simulink model "best_project_for_IG"  (R2023a)
settings: Solver=VariableStepAuto  StartTime=0.0  StopTime=t_final  RelTol=1e-3
StopFcn:
  | generateIndividualReport
values from neighbouring files (symbols this model uses):
  dq_0 = [0; 0; 0]    [Initialization.m]
  dt = 1.00e-03    (= 0.001)    [Initialization.m]
  initPosition = FwdKin(q_0)    [defineTrajectory.m]
undefined symbols (not defined in the file or in its folder): ikInitGuessSim, P1_R1_waypoints, P1_R1_waypointTimes, P1_R1_waypointVels, P2_R2_waypoints
libraries: simulink x6, robotcorelib x4, robotmaniplib x2
settings Model: Creator=lukasz  LastModifiedBy=lukasz

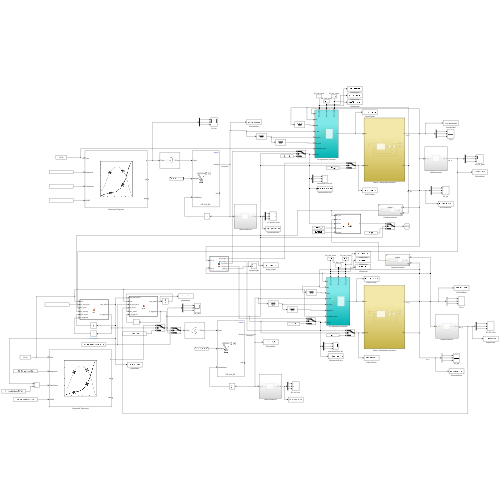
[thumbnail: Simulink's stored preview of the top-level diagram]
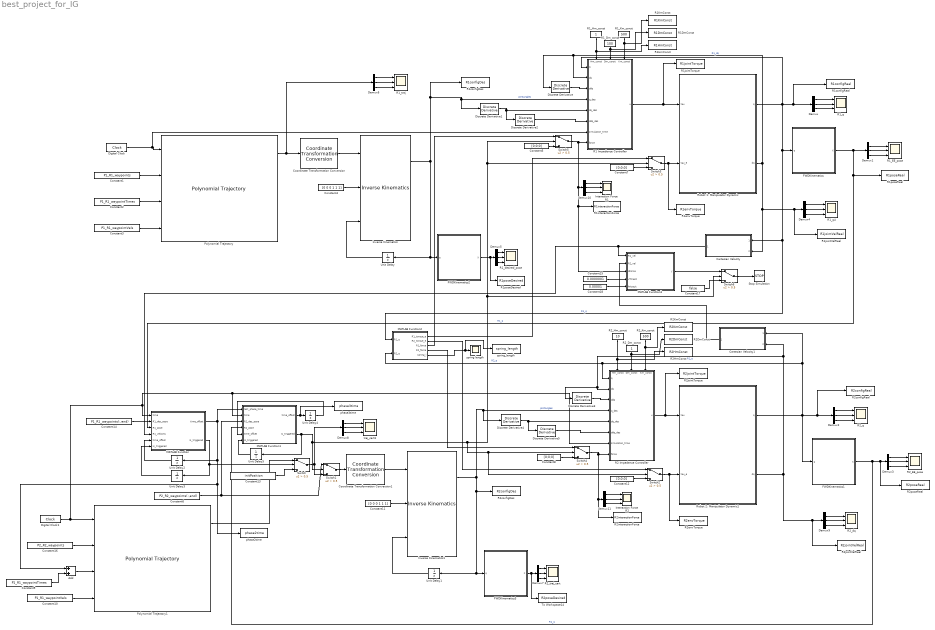
== system best_project_for_IG ==
  Add : Sum
  Cartesian Velocity : Subsystem  ReferencedSubsystem=dq2dp
  Cartesian Velocity1 : Subsystem  ReferencedSubsystem=dq2dp
  Constant1 : Constant  Value=P1_R1_waypoints  VectorParams1D=off  SampleTime=-1
  Constant10 : Constant  Value=P1_R1_waypointVels  VectorParams1D=off  SampleTime=-1
  Constant11 : Constant  Value=[0 0 0 1 1 1]  VectorParams1D=off
  Constant{5,7..8,12} (4 alike) : Constant  Value=[0;0;0]  VectorParams1D=off  SampleTime=-1
  Constant13 : Constant  Value=initPosition  VectorParams1D=off  SampleTime=-1
  Constant14 : Constant  Value=P1_R1_waypoints(:,end)  VectorParams1D=off  SampleTime=-1
  Constant15 : Constant  Value=0.0000001  VectorParams1D=off  SampleTime=-1
  Constant16 : Constant  Value=P2_R2_waypoints  VectorParams1D=off  SampleTime=-1
  Constant17 : Constant  Value=false  VectorParams1D=off  SampleTime=-1
  Constant18 : Constant  Value=0.00001  VectorParams1D=off  SampleTime=-1
  Constant2 : Constant  Value=P1_R1_waypointTimes  VectorParams1D=off  SampleTime=-1
  Constant3 : Constant  Value=P1_R1_waypointVels  VectorParams1D=off  SampleTime=-1
  Constant4 : Constant  Value=[0 0 0 1 1 1]  VectorParams1D=off
  Constant6 : Constant  Value=P2_R2_waypoints(:,end)  VectorParams1D=off  SampleTime=-1
  Constant9 : Constant  Value=P1_R1_waypointTimes  VectorParams1D=off  SampleTime=-1
  Coordinate Transformation Conversion : robotcorelib/Coordinate Transformation Conversion  InputRepresentation=Translation Vector  InputEulerSequence=ZYX  ShowTrVecInputPort=on  OutputRepresentation=Homogeneous Transformation  OutputEulerSequence=ZYX  ShowTrVecOutputPort=on  SimulateUsing=Code generation
  Coordinate Transformation Conversion1 : robotcorelib/Coordinate Transformation Conversion  InputRepresentation=Translation Vector  InputEulerSequence=ZYX  ShowTrVecInputPort=on  OutputRepresentation=Homogeneous Transformation  OutputEulerSequence=ZYX  ShowTrVecOutputPort=on  SimulateUsing=Code generation
  Demux{,1..11} (12 alike) : Demux  Outputs=3
  Digital Clock : DigitalClock  SampleTime=dt
  Digital Clock1 : DigitalClock  SampleTime=dt
  Discrete Derivative{,1..5} (6 alike) : simulink/Discrete/Discrete Derivative  gainval=1.0  ICPrevScaledInput=1  OutMin=[]  OutMax=[]  OutDataType=fixdt(1, 16)  OutScaling=2^-10  DoSatur=off
  FWDKinematics : Subsystem
  FWDKinematics1 : Subsystem
  FWDKinematics2 : Subsystem
  FWDKinematics3 : Subsystem
  Interaction Force R1 : Scope  NumInputPorts=3
  Interaction Force R2 : Scope  NumInputPorts=3
  Inverse Kinematics : robotmaniplib/Inverse Kinematics  RigidBodyTree=robot1  EndEffector=Link_EE  ShowInfo=on  SolverName=BFGS Gradient Projection  EnforceJointLimits=on  MaxIterations=1500  MaxTime=10  GradientTolerance=1e-7  SolutionTolerance=1e-6  StepTolerance=1e-14  ErrorChangeTolerance=1e-12  UseErrorDamping=on  DampingBias=0.0025  SimulateUsing=Code generation
  Inverse Kinematics1 : robotmaniplib/Inverse Kinematics  RigidBodyTree=robot1  EndEffector=Link_EE  ShowInfo=on  SolverName=BFGS Gradient Projection  EnforceJointLimits=on  MaxIterations=1500  MaxTime=10  GradientTolerance=1e-7  SolutionTolerance=1e-6  StepTolerance=1e-14  ErrorChangeTolerance=1e-12  UseErrorDamping=on  DampingBias=0.0025  SimulateUsing=Code generation
  MATLAB Function : MATLAB Function  TreatAsAtomicUnit=on
  MATLAB Function1 : MATLAB Function  TreatAsAtomicUnit=on
  MATLAB Function2 : MATLAB Function  TreatAsAtomicUnit=on
  MATLAB Function3 : MATLAB Function  TreatAsAtomicUnit=on
  Polynomial Trajectory : robotcorelib/Polynomial Trajectory  WaypointSource=External  Waypoints=[ 0, 2, 1, 5, 0; -1, 3, 1, 4, 4 ]  TimePoints=[ 0, 1, 2, 3, 4 ]  TimeInterval=[ 1, 4 ]  Method=Cubic Polynomial  ParameterSource=External  VelocityBoundaryCondition=zeros( 2, 5 )  AccelerationBoundaryCondition=zeros( 2, 5 )  SimulateUsing=Interpreted execution
  Polynomial Trajectory1 : robotcorelib/Polynomial Trajectory  WaypointSource=External  Waypoints=[ 0, 2, 1, 5, 0; -1, 3, 1, 4, 4 ]  TimePoints=[ 0, 1, 2, 3, 4 ]  TimeInterval=[ 1, 4 ]  Method=Cubic Polynomial  ParameterSource=External  VelocityBoundaryCondition=zeros( 2, 5 )  AccelerationBoundaryCondition=zeros( 2, 5 )  SimulateUsing=Interpreted execution
  R1 Impedence Controller : Subsystem
      settings: PortSchema="{\"entries\":[{\"content\":{\"sides\":[{\"content\":{\"connectorIds\":[\"In1\",\"In2\",\"In3\",\"In4\",\"In5\",\"In6\",\"In7\",\"In8\"]},\"type\":\"ConnectorPlacement.EquallySpacedRectSide\",\"uuid\":\"5dfe44b3-09a5-4539-84d6-5f1c3b4c2f7b\"},{\"content\":{\"connectorIds\":[\"Out1\"],\"side\":\"RIGHT\"},\"type\":\"ConnectorPlacement.EquallySpacedRectSide\",\"uuid\":\"14568bd5-ea33-4e20-b738-babf2c0b76a3\"},{\"content\":{\"connectorIds\":[\"In9\",\"In10\",\"In11\"],\"side\":\"TOP\"},\"type\":\"ConnectorPlacement.EquallySpacedRectSide\",\"uuid\":\"79ac3c01-1ab3-40ba-b47a-1253ed034708\"}]},\"type\":\"ConnectorPlacement.EquallySpacedConnector\",\"uuid\":\"3e0c5e05-24f3-4436-a36d-058567bfa2f1\"}],\"packageUris\":[\"http://schema.mathworks.com/mf0/Connector/R2020b\"],\"version\":\"1.0\"}"
  R1DmConst : ToWorkspace  VariableName=R1DmConst  SaveFormat=Timeseries  SampleTime=-1
  R1HmConst : ToWorkspace  VariableName=R1HmConst  SaveFormat=Timeseries  SampleTime=-1
  R1KmConst : ToWorkspace  VariableName=R1KmConst  SaveFormat=Timeseries  SampleTime=-1
  R1_Dm_const : Constant  Value=100  VectorParams1D=off  SampleTime=-1
  R1_EE_pose : Scope  NumInputPorts=3
  R1_Hm_const : Constant  VectorParams1D=off  SampleTime=-1
  R1_Km_const : Constant  Value=500  VectorParams1D=off  SampleTime=-1
  R1_desired_pose : Scope  NumInputPorts=3
  R1_q : Scope  NumInputPorts=3
  R1_q4 : Scope  NumInputPorts=3
  R1_traj : Scope  NumInputPorts=3
  R1configDes : ToWorkspace  VariableName=R1configDes  SaveFormat=Timeseries  SampleTime=-1
  R1configReal : ToWorkspace  VariableName=R1configReal  SaveFormat=Timeseries  SampleTime=-1
  R1envTorque : ToWorkspace  VariableName=R1envTorque  SaveFormat=Timeseries  SampleTime=-1
  R1interactionForce : ToWorkspace  VariableName=R1interactionForce  SaveFormat=Timeseries  SampleTime=-1
  R1jointTorque : ToWorkspace  VariableName=R1jointTorque  SaveFormat=Timeseries  SampleTime=-1
  R1jointVelReal : ToWorkspace  VariableName=R1jointVelReal  SaveFormat=Timeseries  SampleTime=-1
  R1poseDesired : ToWorkspace  VariableName=R1poseDesired  SaveFormat=Timeseries  SampleTime=-1
  R1poseReal : ToWorkspace  VariableName=R1poseReal  SaveFormat=Timeseries  SampleTime=-1
  R2 Impedence Controller : Subsystem
      settings: PortSchema="{\"entries\":[{\"content\":{\"sides\":[{\"content\":{\"connectorIds\":[\"In1\",\"In2\",\"In3\",\"In4\",\"In5\",\"In6\",\"In7\",\"In8\"]},\"type\":\"ConnectorPlacement.EquallySpacedRectSide\",\"uuid\":\"5dfe44b3-09a5-4539-84d6-5f1c3b4c2f7b\"},{\"content\":{\"connectorIds\":[\"Out1\"],\"side\":\"RIGHT\"},\"type\":\"ConnectorPlacement.EquallySpacedRectSide\",\"uuid\":\"14568bd5-ea33-4e20-b738-babf2c0b76a3\"},{\"content\":{\"connectorIds\":[\"In9\",\"In10\",\"In11\"],\"side\":\"TOP\"},\"type\":\"ConnectorPlacement.EquallySpacedRectSide\",\"uuid\":\"79ac3c01-1ab3-40ba-b47a-1253ed034708\"}]},\"type\":\"ConnectorPlacement.EquallySpacedConnector\",\"uuid\":\"3e0c5e05-24f3-4436-a36d-058567bfa2f1\"}],\"packageUris\":[\"http://schema.mathworks.com/mf0/Connector/R2020b\"],\"version\":\"1.0\"}"
  R2DmConst : ToWorkspace  VariableName=R2DmConst  SaveFormat=Timeseries  SampleTime=-1
  R2HmConst : ToWorkspace  VariableName=R2HmConst  SaveFormat=Timeseries  SampleTime=-1
  R2KmConst : ToWorkspace  VariableName=R2KmConst  SaveFormat=Timeseries  SampleTime=-1
  R2_Dm_const : Constant  VectorParams1D=off  SampleTime=-1
  R2_EE_pose : Scope  NumInputPorts=3
  R2_Hm_const : Constant  Value=10  VectorParams1D=off  SampleTime=-1
  R2_Km_const : Constant  Value=500  VectorParams1D=off  SampleTime=-1
  R2_dq : Scope  NumInputPorts=3
  R2_q : Scope  NumInputPorts=3
  R2_traj_cart : Scope  NumInputPorts=3
  R2configDes : ToWorkspace  VariableName=R2configDes  SaveFormat=Timeseries  SampleTime=-1
  R2configReal : ToWorkspace  VariableName=R2configReal  SaveFormat=Timeseries  SampleTime=-1
  R2envTorque : ToWorkspace  VariableName=R2envTorque  SaveFormat=Timeseries  SampleTime=-1
  R2interactionForce : ToWorkspace  VariableName=R2interactionForce  SaveFormat=Timeseries  SampleTime=-1
  R2jointTorque : ToWorkspace  VariableName=R2jointTorque  SaveFormat=Timeseries  SampleTime=-1
  R2jointVelReal : ToWorkspace  VariableName=R2jointVelReal  SaveFormat=Timeseries  SampleTime=-1
  R2poseReal : ToWorkspace  VariableName=R2poseReal  SaveFormat=Timeseries  SampleTime=-1
  Robot 1: Manipulator Dynamic : Subsystem
  Robot 2: Manipulator Dynamic1 : Subsystem
  Stop Simulation : Stop
  Switch{,1..6} (7 alike) : Switch  Criteria=u2 > Threshold  Threshold=0.5  SaturateOnIntegerOverflow=off  InputSameDT=off
  To Workspace14 : ToWorkspace  VariableName=R2poseDesired  SaveFormat=Timeseries  SampleTime=-1
  Unit Delay : UnitDelay  InitialCondition=ikInitGuessSim  SampleTime=-1  HasFrameUpgradeWarning=on
  Unit Delay1 : UnitDelay  InitialCondition=ikInitGuessSim  SampleTime=-1  HasFrameUpgradeWarning=on
  Unit Delay{2..5} (4 alike) : UnitDelay  SampleTime=-1  HasFrameUpgradeWarning=on
  phase2time : ToWorkspace  VariableName=phase2time  SaveFormat=Timeseries  SampleTime=-1
  phase3time : ToWorkspace  VariableName=phase3time  SaveFormat=Timeseries  SampleTime=-1
  spring length : Scope
  spring_length : ToWorkspace  VariableName=spring_length  SaveFormat=Timeseries  SampleTime=-1
  traj_cart3 : Scope  NumInputPorts=3
  wires:
  Demux/3 -> R1_q/3
  Robot 1: Manipulator Dynamic/1(q) -> R1 Impedence Controller/1(q), FWDKinematics/1(q), MATLAB Function2/1(R1_q), Cartesian Velocity/1, R1configReal/1, Demux/1  "R1_q"
  Demux/1 -> R1_q/1
  Demux/2 -> R1_q/2
  Constant1/1 -> Polynomial Trajectory/2
  Inverse Kinematics/1 -> FWDKinematics2/1(q), Unit Delay/1, R1configDes/1, Discrete Derivative1/1, R1 Impedence Controller/4(q_des)  "jointAngles"
  Unit Delay/1 -> Inverse Kinematics/3
  Constant4/1 -> Inverse Kinematics/2
  Digital Clock/1 -> R1 Impedence Controller/7(simulation_time), Polynomial Trajectory/1
  Constant3/1 -> Polynomial Trajectory/4
  Constant2/1 -> Polynomial Trajectory/3
  Demux1/1 -> R1_EE_pose/1
  Demux1/2 -> R1_EE_pose/2
  Demux1/3 -> R1_EE_pose/3
  FWDKinematics/1(X) -> R1poseReal/1, MATLAB Function/3(R1_pose), Demux1/1  "R1_q"
  Demux3/2 -> R2_EE_pose/2
  Demux2/3 -> R2_q/3
  Demux3/1 -> R2_EE_pose/1
  Demux2/1 -> R2_q/1
  Demux2/2 -> R2_q/2
  Demux3/3 -> R2_EE_pose/3
  Robot 2: Manipulator Dynamic1/1(q) -> Cartesian Velocity1/1, R2 Impedence Controller/1(q), MATLAB Function2/2(R2_q), FWDKinematics1/1(q), R2configReal/1, Demux2/1  "R2_q"
  FWDKinematics1/1(X) -> MATLAB Function1/4(R2_pose), R2poseReal/1, Demux3/1  "R1_q"
  Demux4/1 -> R1_q4/1
  Demux4/2 -> R1_q4/2
  Demux4/3 -> R1_q4/3
  Robot 1: Manipulator Dynamic/2(dq) -> Discrete Derivative/1, R1 Impedence Controller/2(dq), Cartesian Velocity/2, R1jointVelReal/1, Demux4/1  "R1_dq"
  Demux5/1 -> R1_desired_pose/1
  Demux5/2 -> R1_desired_pose/2
  Demux5/3 -> R1_desired_pose/3
  FWDKinematics2/1(X) -> R1poseDesired/1, Demux5/1
  Demux6/3 -> R1_traj/3
  Demux6/1 -> R1_traj/1
  Demux6/2 -> R1_traj/2
  Polynomial Trajectory/1 -> Coordinate Transformation Conversion/1, Demux6/1
  Coordinate Transformation Conversion/1 -> Inverse Kinematics/1
  R1 Impedence Controller/1(u) -> R1jointTorque/1, Robot 1: Manipulator Dynamic/1(tau)
  Discrete Derivative/1 -> R1 Impedence Controller/3(ddq)
  Discrete Derivative1/1 -> Discrete Derivative2/1, R1 Impedence Controller/5(dq_des)
  Discrete Derivative2/1 -> R1 Impedence Controller/6(ddq_des)
  Unit Delay1/1 -> Inverse Kinematics1/3
  Digital Clock1/1 -> MATLAB Function/1(time), R2 Impedence Controller/7(simulation_time), MATLAB Function1/2(time), Polynomial Trajectory1/1
  Demux7/1 -> R2_traj_cart/1
  Discrete Derivative4/1 -> R2 Impedence Controller/5(dq_des), Discrete Derivative5/1
  Constant16/1 -> Polynomial Trajectory1/2
  Inverse Kinematics1/1 -> R2configDes/1, FWDKinematics3/1(q), Unit Delay1/1, R2 Impedence Controller/4(q_des), Discrete Derivative4/1  "jointAngles"
  Discrete Derivative5/1 -> R2 Impedence Controller/6(ddq_des)
  Demux7/3 -> R2_traj_cart/3
  R2 Impedence Controller/1(u) -> R2jointTorque/1, Robot 2: Manipulator Dynamic1/1(tau)
  Demux7/2 -> R2_traj_cart/2
  FWDKinematics3/1(X) -> To Workspace14/1, Demux7/1
  Discrete Derivative3/1 -> R2 Impedence Controller/3(ddq)
  Demux8/3 -> traj_cart3/3
  Demux8/2 -> traj_cart3/2
  Constant11/1 -> Inverse Kinematics1/2
  Constant10/1 -> Polynomial Trajectory1/4
  Demux8/1 -> traj_cart3/1
  Coordinate Transformation Conversion1/1 -> Inverse Kinematics1/1
  Demux9/3 -> R2_dq/3
  Demux9/1 -> R2_dq/1
  Robot 2: Manipulator Dynamic1/2(dq) -> R2jointVelReal/1, Demux9/1, R2 Impedence Controller/2(dq), Discrete Derivative3/1, Cartesian Velocity1/2  "R1_q"
  Demux9/2 -> R2_dq/2
  Switch/1 -> Switch1/3, Demux8/1
  Polynomial Trajectory1/1 -> Switch/1
  Constant13/1 -> Switch/3
  Unit Delay2/1 -> MATLAB Function/5("time_offset ")
  Add/1 -> Polynomial Trajectory1/3
  Constant9/1 -> Add/2
  Unit Delay3/1 -> MATLAB Function/6("is_triggered ")
  MATLAB Function/2(is_triggered) -> Switch/2, Unit Delay3/1
  MATLAB Function/1(time_offset) -> phase2time/1, Add/1, Unit Delay2/1, MATLAB Function1/1(last_phase_time)
  Constant14/1 -> MATLAB Function/2(R1_des_pose)
  Cartesian Velocity/1 -> MATLAB Function/4(R1_velocity), MATLAB Function3/1(R1_vel)
  Switch1/1 -> Coordinate Transformation Conversion1/1
  MATLAB Function1/2(is_triggered) -> Unit Delay5/1, Switch5/2, Switch3/2, Switch6/2, Switch2/2, Switch4/2, Switch1/2
  MATLAB Function1/1(time_offset) -> phase3time/1, Unit Delay4/1
  Unit Delay4/1 -> MATLAB Function1/5("time_offset ")
  Unit Delay5/1 -> MATLAB Function1/6("is_triggered ")
  Constant6/1 -> Switch1/1, MATLAB Function1/3(R2_des_pose)
  Switch2/1 -> R2envTorque/1, Robot 2: Manipulator Dynamic1/2(tau_e)
  Switch3/1 -> R1envTorque/1, Robot 1: Manipulator Dynamic/2(tau_e)
  Constant5/1 -> Switch5/3
  Constant7/1 -> Switch3/3
  Constant8/1 -> Switch4/3
  Constant12/1 -> Switch2/3
  MATLAB Function2/4(R2_force) -> Switch4/1
  MATLAB Function2/2(R2_torque_e) -> Switch2/1
  MATLAB Function2/1(R1_torque_e) -> Switch3/1
  MATLAB Function2/3(R1_force) -> Switch5/1
  Demux10/1 -> Interaction Force R1/1
  Demux10/2 -> Interaction Force R1/2
  Demux10/3 -> Interaction Force R1/3
  Switch5/1 -> MATLAB Function3/3(dForce), R1interactionForce/1, Demux10/1, R1 Impedence Controller/8(force)
  Demux11/3 -> Interaction Force R2/3
  Demux11/1 -> Interaction Force R2/1
  Switch4/1 -> R2 Impedence Controller/8(force), R2interactionForce/1, Demux11/1
  Demux11/2 -> Interaction Force R2/2
  MATLAB Function2/5(spring_l) -> spring_length/1, spring length/1
  R1_Hm_const/1 -> R1 Impedence Controller/9(Hm_const), R1HmConst/1
  R1_Dm_const/1 -> R1 Impedence Controller/10(Dm_const), R1DmConst/1
  R1_Km_const/1 -> R1 Impedence Controller/11(Km_const), R1KmConst/1
  R2_Km_const/1 -> R2KmConst/1, R2 Impedence Controller/11(Km_const)
  R2_Hm_const/1 -> R2HmConst/1, R2 Impedence Controller/9(Hm_const)
  R2_Dm_const/1 -> R2 Impedence Controller/10(Dm_const), R2DmConst/1
  MATLAB Function3/1(y) -> Switch6/1
  Switch6/1 -> Stop Simulation/1
  Constant17/1 -> Switch6/3
  Cartesian Velocity1/1 -> MATLAB Function3/2(R2_vel)
  Constant15/1 -> MATLAB Function3/4(vThresh)
  Constant18/1 -> MATLAB Function3/5(fThresh)

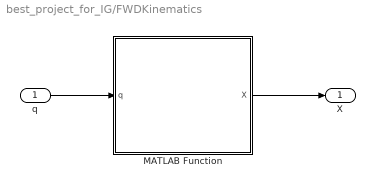
== system best_project_for_IG/FWDKinematics ==
  q : Inport
  MATLAB Function : MATLAB Function  TreatAsAtomicUnit=on
  X : Outport
  wires:
  MATLAB Function/1(X) -> X/1
  q/1 -> MATLAB Function/1(q)

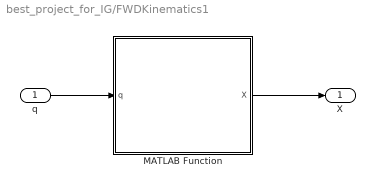
== system best_project_for_IG/FWDKinematics1 ==
  q : Inport
  MATLAB Function : MATLAB Function  TreatAsAtomicUnit=on
  X : Outport
  wires:
  MATLAB Function/1(X) -> X/1
  q/1 -> MATLAB Function/1(q)

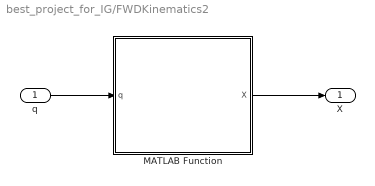
== system best_project_for_IG/FWDKinematics2 ==
  q : Inport
  MATLAB Function : MATLAB Function  TreatAsAtomicUnit=on
  X : Outport
  wires:
  MATLAB Function/1(X) -> X/1
  q/1 -> MATLAB Function/1(q)

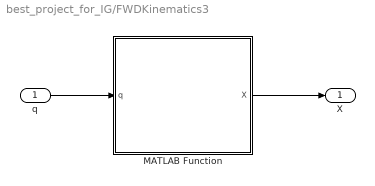
== system best_project_for_IG/FWDKinematics3 ==
  q : Inport
  MATLAB Function : MATLAB Function  TreatAsAtomicUnit=on
  X : Outport
  wires:
  MATLAB Function/1(X) -> X/1
  q/1 -> MATLAB Function/1(q)

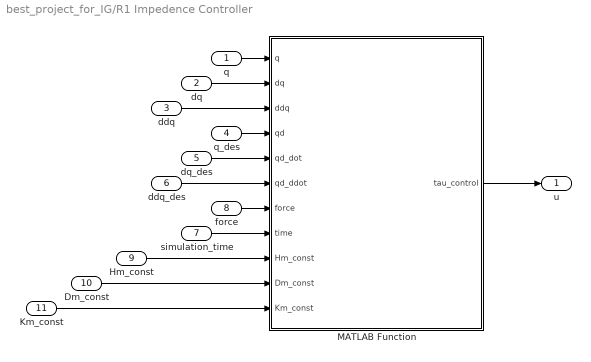
== system best_project_for_IG/R1 Impedence Controller ==
  q : Inport
  dq : Inport  Port=2
  ddq : Inport  Port=3
  q_des : Inport  Port=4
  dq_des : Inport  Port=5
  ddq_des : Inport  Port=6
  simulation_time : Inport  Port=7
  force : Inport  Port=8
  Hm_const : Inport  Port=9
  Dm_const : Inport  Port=10
  Km_const : Inport  Port=11
  MATLAB Function : MATLAB Function  TreatAsAtomicUnit=on
  u : Outport
  wires:
  dq/1 -> MATLAB Function/2(dq)
  MATLAB Function/1(tau_control) -> u/1
  q_des/1 -> MATLAB Function/4(qd)
  q/1 -> MATLAB Function/1(q)
  ddq_des/1 -> MATLAB Function/6(qd_ddot)
  dq_des/1 -> MATLAB Function/5(qd_dot)
  simulation_time/1 -> MATLAB Function/8(time)
  ddq/1 -> MATLAB Function/3(ddq)
  force/1 -> MATLAB Function/7(force)
  Hm_const/1 -> MATLAB Function/9(Hm_const)
  Dm_const/1 -> MATLAB Function/10(Dm_const)
  Km_const/1 -> MATLAB Function/11(Km_const)

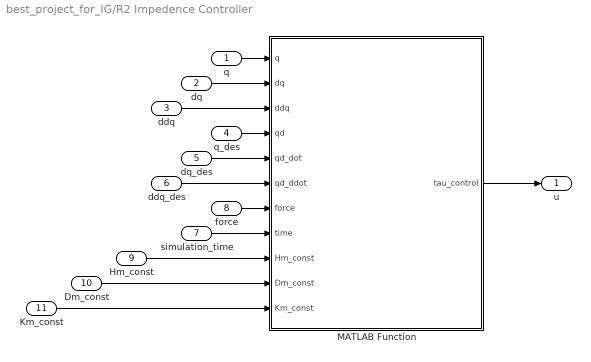
== system best_project_for_IG/R2 Impedence Controller ==
  q : Inport
  dq : Inport  Port=2
  ddq : Inport  Port=3
  q_des : Inport  Port=4
  dq_des : Inport  Port=5
  ddq_des : Inport  Port=6
  simulation_time : Inport  Port=7
  force : Inport  Port=8
  Hm_const : Inport  Port=9
  Dm_const : Inport  Port=10
  Km_const : Inport  Port=11
  MATLAB Function : MATLAB Function  TreatAsAtomicUnit=on
  u : Outport
  wires:
  dq/1 -> MATLAB Function/2(dq)
  MATLAB Function/1(tau_control) -> u/1
  q_des/1 -> MATLAB Function/4(qd)
  q/1 -> MATLAB Function/1(q)
  ddq_des/1 -> MATLAB Function/6(qd_ddot)
  dq_des/1 -> MATLAB Function/5(qd_dot)
  simulation_time/1 -> MATLAB Function/8(time)
  ddq/1 -> MATLAB Function/3(ddq)
  force/1 -> MATLAB Function/7(force)
  Hm_const/1 -> MATLAB Function/9(Hm_const)
  Dm_const/1 -> MATLAB Function/10(Dm_const)
  Km_const/1 -> MATLAB Function/11(Km_const)

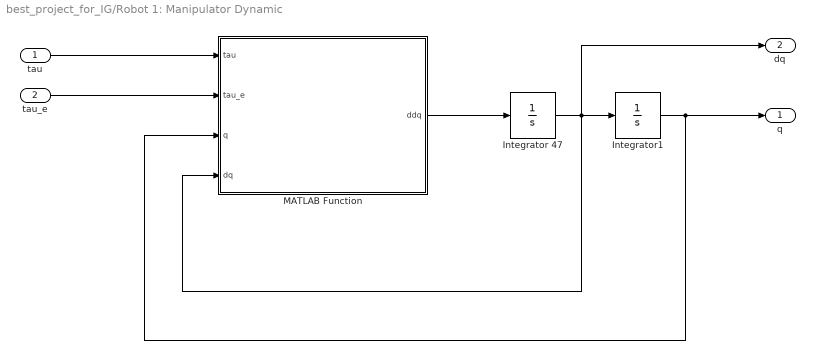
== system best_project_for_IG/Robot 1: Manipulator Dynamic ==
  tau : Inport
  tau_e : Inport  Port=2
  Integrator 47 : Integrator  InitialCondition=dq_0
  Integrator1 : Integrator  InitialCondition=ikInitGuessSim
  MATLAB Function : MATLAB Function  TreatAsAtomicUnit=on
  q : Outport
  dq : Outport  Port=2
  wires:
  MATLAB Function/1(ddq) -> Integrator 47/1
  tau/1 -> MATLAB Function/1(tau)
  tau_e/1 -> MATLAB Function/2(tau_e)
  Integrator1/1 -> q/1, MATLAB Function/3(q)
  Integrator 47/1 -> dq/1, MATLAB Function/4(dq), Integrator1/1

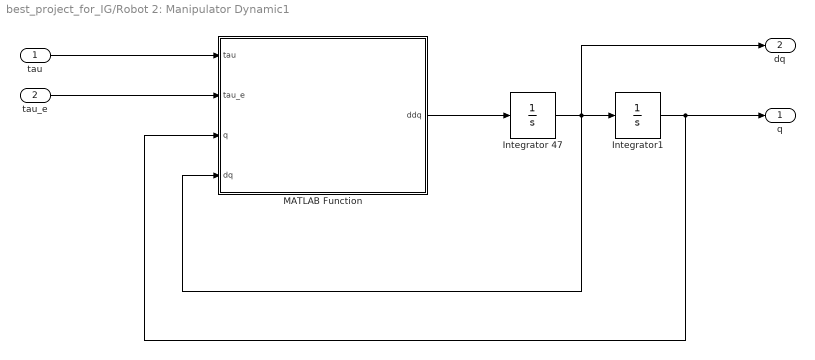
== system best_project_for_IG/Robot 2: Manipulator Dynamic1 ==
  tau : Inport
  tau_e : Inport  Port=2
  Integrator 47 : Integrator  InitialCondition=dq_0
  Integrator1 : Integrator  InitialCondition=ikInitGuessSim
  MATLAB Function : MATLAB Function  TreatAsAtomicUnit=on
  q : Outport
  dq : Outport  Port=2
  wires:
  MATLAB Function/1(ddq) -> Integrator 47/1
  tau/1 -> MATLAB Function/1(tau)
  tau_e/1 -> MATLAB Function/2(tau_e)
  Integrator1/1 -> q/1, MATLAB Function/3(q)
  Integrator 47/1 -> dq/1, MATLAB Function/4(dq), Integrator1/1

== matlab function best_project_for_IG/MATLAB Function1 ==
  data: last_phase_time input; time input; R2_des_pose input; R2_pose input; time_offset input; time_offset output; is_triggered input; is_triggered output
function [time_offset, is_triggered] = fcn(last_phase_time, time, R2_des_pose, R2_pose, time_offset, is_triggered)

x_trigger = R2_des_pose(1);
current_x = R2_pose(1);

if ((time > (last_phase_time+6)) && ...
        current_x >= x_trigger && (is_triggered==0))
    time_offset = time;
    is_triggered = 1;
end

== matlab function best_project_for_IG/R1 Impedence Controller/MATLAB Function ==
  data: q input; dq input; ddq input; tau_control output; qd input; qd_dot input; qd_ddot input; force input; time input; Hm_const input; Dm_const input; Km_const input
function tau_control = fcn(q, dq, ddq, qd, qd_dot, qd_ddot,force,...
                           time, Hm_const, Dm_const, Km_const)
% reset first qd_ddot
if (time < 0.003)
    qd_ddot = [0;0;0];
    qd_dot = [0;0;0];
    ddq = [0;0;0];
end


%% Joint Space variables

q1 = q(1);
q2 = q(2);
q3 = q(3);

dq1 = dq(1);
dq2 = dq(2);
dq3 = dq(3);

%% general physical parameters

l1 = 0.6731;
l2 = 0.432;
l3 = 0.434;
lc2 = 0.216;
lc3 = 0.164;
m2 = 15.46;
m3 = 9.55;
J = 0.302;

%% Inertia Matrix Parameters

J1 = m3 * lc3^2;
J12 = (m2 * lc2^2) + (m3 * l2^2);
J13 = l2 * lc3 * m3;


h11 = J + J1 * (sin(q2 + q3))^2 + J12 * (cos(q2))^2 + 2 * J13 * cos(q2) * sin(q2+q3);
h22 = J1 + J12 + 2 * J13 * sin(q3);
h23 = J1 + J13 * sin(q3);
h32 = h23;
h33 = J1;

H = [h11, 0 ,0 ;
    0 , h22, h23;
    0 , h32, h33];

%% Coriolis Matrix Parameters

c12_1 = J1 * sin(2 * (q1 + q2)) - J12 * sin(2 * q2) + 2 * J13 * cos(2 * q2 +q3);
c13_1 = J1 * sin(2 * (q2 + q3)) + 2 * J13 * cos(q2) * cos(q2 + q3);
c11_2 = (1/2) * (-J1 * sin(2 * (q2 + q3)) + J12 * sin(2 * q2) - 2 * J13 * cos(2 * q2 + q3));
c22_2 = 2 * J13 * cos(q3);
c23_2 = J13 * cos(q3);
c22_3 = -J13 * cos(q3) * dq2;
c11_3 = (-1/2) * (J1 * sin(2 * (q2 + q3)) + J13 * cos(q2) * cos(q2 + q3));

C = [0, c12_1 * dq1, c13_1 * dq3;
    c11_2 * dq1, 0 , c22_2 * dq2 + c23_2 * dq3;
    c11_3 * dq1, c22_3 * dq2, 0];

%% Vector of Potential Forces Parameters

g = 9.81;

g21 = -g * (lc3 * m3 * sin(q2 + q3) + lc2 * m2 * cos(q2) + l2 * m3 * cos(q2));
g31 = -g * (lc3 * m3 * sin(q2 + q3));

G = [0;
    g21;
    g31];


%% get Jacobians
J = jacobian(q);
dJ = dJacobian(q,dq);

%% convert to task space
Hp = inv(J') * H * inv(J);
Cp = inv(J') * C * inv(J) - Hp * dJ * inv(J);
Gp = inv(J') * G;

%% desired behaviour
Hm = Hm_const*eye(3,3);
Dm = Dm_const*eye(3,3);
Km = Km_const*eye(3,3);

%% get postion and its derivs
p = fwdKin(q);
dp = J * dq;
ddp = dJ * dq + J * ddq;

%% get desired postion and its derivs
pd = fwdKin(qd);
pd_dot = jacobian(qd) * qd_dot;
pd_ddot = dJacobian(qd,qd_dot) * qd_dot + jacobian(qd) * qd_ddot;

%% define u note

u_note = pd_ddot + inv(Hm) * (Dm * (pd_dot-dp) + Km*(pd - p) + force);
inv_hm = inv(Hm);
%% define tau_control

tau_control = J' * (Hp * u_note + Cp * dp + Gp - force);


function [X] = fwdKin(Q)
    s1 = sin(Q(1, :));
    c1 = cos(Q(1, :));
    s2 = sin(Q(2, :));
    c2 = cos(Q(2, :));
    s23 = sin(Q(2, :) + Q(3, :));
    c23 = cos(Q(2, :) + Q(3, :));
    l = [0.6731; 0.432; 0.434];
    
    X = zeros(3,1);
    X(1, :) = c1.*(l(2)*c2 + l(3)*s23);
    X(2, :) = s1.*(l(2)*c2 + l(3)*s23);
    X(3, :) = l(1) - l(2)*s2 + l(3)*c23;

function dJ = dJacobian(Q, dQ)
    l = [0.6731; 0.432; 0.434];
    s1 = sin(Q(1));
    c1 = cos(Q(1));
    s2 = sin(Q(2));
    c2 = cos(Q(2));
    s23 = sin(Q(2) + Q(3));
    c23 = cos(Q(2) + Q(3));

    % dJi derivative of each element of Jacobian wrt i-th variable            
    %--- 1 ---
    dJ1 = [-c1*(l(2)*c2 + l(3)*s23), -s1*(-l(2)*s2 + l(3)*c23), -l(3)*s1*c23;...
           -s1*(l(2)*c2 + l(3)*s23),  c1*(-l(2)*s2 + l(3)*c23),  l(3)*c1*c23;...
           0, 0, 0];
    %--- 2 ---   
    dJ2 = [-s1*(-l(2)*s2 + l(3)*c23), -c1*(l(2)*c2 + l(3)*s23), -l(3)*c1*s23;...
            c1*(-l(2)*s2 + l(3)*c23), -s1*(l(2)*c2 + l(3)*s23), -l(3)*s1*s23;...
            0, l(2)*s2 - l(3)*c23, -l(3)*c23];

    %--- 3 ---
    dJ3 = -l(3)*[ s1*c23, c1*s23, c1*s23;...
                 -c1*c23, s1*s23, s1*s23;...
                 0, c23, c23];
    %--- dJ ---
    dJ = dJ1*dQ(1) + dJ2*dQ(2) + dJ3*dQ(3);

function [J] = jacobian(q)

l = [0.6731; 0.432; 0.434];
s1 = sin(q(1));
c1 = cos(q(1));
s2 = sin(q(2));
c2 = cos(q(2));
s23 = sin(q(2) + q(3));
c23 = cos(q(2) + q(3));

J = zeros(3,3);

J(1, 1) = -s1*( l(2)*c2 + l(3)*s23);
J(1, 2) =  c1*(-l(2)*s2 + l(3)*c23);
J(1, 3) = l(3)*c1*c23;

J(2, 1) = c1*( l(2)*c2 + l(3)*s23);
J(2, 2) = s1*(-l(2)*s2 + l(3)*c23);
J(2, 3) = l(3)*s1*c23;

J(3, 2) = -l(2)*c2 - l(3)*s23;
J(3, 3) = -l(3)*s23;

== matlab function best_project_for_IG/MATLAB Function3 ==
  data: R1_vel input; y output; R2_vel input; dForce input; vThresh input; fThresh input
function y = stopCondition(R1_vel, R2_vel, dForce, vThresh, fThresh)

if (norm(R1_vel) <= vThresh) && ...
   (norm(R2_vel) <= vThresh) && ...
   (norm(dForce) <= fThresh)
    y = true;
else
    y = false;
end

end

== matlab function best_project_for_IG/MATLAB Function2 ==
  data: R1_q input; R1_torque_e output; R2_q input; R2_torque_e output; R1_force output; R2_force output; spring_l output
function [R1_torque_e, R2_torque_e, R1_force, R2_force, spring_l] = fcn(R1_q, R2_q)

uncompressed_spring_len = 0.2;

R1_pose = fwdKin(R1_q);
R2_pose = fwdKin(R2_q);

% transforms and rod definition
rod_length = [0.20;0;0]; % meters
R1_T_R2 = [-1,  0,  0, 0.7395*2 + rod_length(1);
            0, -1,  0,                            0;
            0,  0,  1,                            0;
            0,  0,  0,                            1];

R2_T_R1 = [-1,  0,  0, 0.7395*2 + rod_length(1);
            0, -1,  0,                            0;
            0,  0,  1,                            0;
            0,  0,  0,                            1];

R2_pose_in_R1 = R1_T_R2*[R2_pose;1];
R2_pose_in_R1 = R2_pose_in_R1(1:3);



spring_l = norm(R2_pose_in_R1 - R1_pose);
spring_unitVec = (R2_pose_in_R1 - R1_pose)/norm(R2_pose_in_R1 - R1_pose);
compression_d = spring_l-uncompressed_spring_len; % positive is strech

k = 500;


R1_force = k * compression_d * spring_unitVec;
R2_force = R2_T_R1(1:3,1:3)*-R1_force;
R2_force = R2_force(1:3);

R1_jacobian = jacobian(R1_q);
R2_jacobian = jacobian(R2_q);

R1_torque_e = R1_jacobian'*R1_force;
R2_torque_e = R2_jacobian'*R2_force;

function [X] = fwdKin(Q)
    s1 = sin(Q(1, :));
    c1 = cos(Q(1, :));
    s2 = sin(Q(2, :));
    c2 = cos(Q(2, :));
    s23 = sin(Q(2, :) + Q(3, :));
    c23 = cos(Q(2, :) + Q(3, :));
    l = [0.6731; 0.432; 0.434];
    
    X = zeros(3,1);
    X(1, :) = c1.*(l(2)*c2 + l(3)*s23);
    X(2, :) = s1.*(l(2)*c2 + l(3)*s23);
    X(3, :) = l(1) - l(2)*s2 + l(3)*c23;

function [J] = jacobian(q)

l = [0.6731; 0.432; 0.434];
s1 = sin(q(1));
c1 = cos(q(1));
s2 = sin(q(2));
c2 = cos(q(2));
s23 = sin(q(2) + q(3));
c23 = cos(q(2) + q(3));

J = zeros(3,3);

J(1, 1) = -s1*( l(2)*c2 + l(3)*s23);
J(1, 2) =  c1*(-l(2)*s2 + l(3)*c23);
J(1, 3) = l(3)*c1*c23;

J(2, 1) = c1*( l(2)*c2 + l(3)*s23);
J(2, 2) = s1*(-l(2)*s2 + l(3)*c23);
J(2, 3) = l(3)*s1*c23;

J(3, 2) = -l(2)*c2 - l(3)*s23;
J(3, 3) = -l(3)*s23;

== matlab function best_project_for_IG/FWDKinematics/MATLAB Function ==
  data: q input; X output
function X = FWDKinematics(q)
%%% Forward Kinematic Function


%% Joint Space variables
% q is 3*1 vector of joint variables (radian), q = [q1;q2;q3]
q1 = q(1);
q2 = q(2);
q3 = q(3);

%% general physical parameters
l1 = 0.6731;
l2 = 0.432;
l3 = 0.434;
lc2 = 0.216;
lc3 = 0.164;

%% Forward Kinematic
% X is 3*1 vecto of end-effector position in task space, X = [x;y;z]

x = cos(q1) * (l2 * cos(q2) + l3 * sin(q2 + q3));
y = sin(q1) * (l2 * cos(q2) + l3 * sin(q2 + q3));
z = l1 - l2 * sin(q2) + l3 * cos(q2 + q3);

X = [x;y;z];

== matlab function best_project_for_IG/FWDKinematics1/MATLAB Function ==
  data: q input; X output
function X = FWDKinematics(q)
%%% Forward Kinematic Function


%% Joint Space variables
% q is 3*1 vector of joint variables (radian), q = [q1;q2;q3]
q1 = q(1);
q2 = q(2);
q3 = q(3);

%% general physical parameters
l1 = 0.6731;
l2 = 0.432;
l3 = 0.434;
lc2 = 0.216;
lc3 = 0.164;

%% Forward Kinematic
% X is 3*1 vecto of end-effector position in task space, X = [x;y;z]

x = cos(q1) * (l2 * cos(q2) + l3 * sin(q2 + q3));
y = sin(q1) * (l2 * cos(q2) + l3 * sin(q2 + q3));
z = l1 - l2 * sin(q2) + l3 * cos(q2 + q3);

X = [x;y;z];

== matlab function best_project_for_IG/Robot 2: Manipulator Dynamic1/MATLAB Function ==
  data: tau input; tau_e input; q input; ddq output; dq input
function ddq = DynamicModel( tau, tau_e, q, dq)
%%%%%
% 3-DOF Puma-560 Dynamic Model Function
% H(q)* ddq + C(q) * dq + G = tau + tau_e
% q is 3*1 vector of joint variables (radian)
% H(q) is the inertia matrix
% C(q) is the matrix of Coriolis and centrifugal forces
% G(q) is  the vector of potential forces Parameters
% tau is control torque 
% tau_e is the external torque due to the interaction with the environment
%%%%%

%% Joint Space variables

q1 = q(1);
q2 = q(2);
q3 = q(3);

dq1 = dq(1);
dq2 = dq(2);
dq3 = dq(3);

%% general physical parameters

l1 = 0.6731;
l2 = 0.432;
l3 = 0.434;
lc2 = 0.216;
lc3 = 0.164;
m2 = 15.46;
m3 = 9.55;
J = 0.302;

%% Inertia Matrix Parameters

J1 = m3 * lc3^2;
J12 = (m2 * lc2^2) + (m3 * l2^2);
J13 = l2 * lc3 * m3;


h11 = J + J1 * (sin(q2 + q3))^2 + J12 * (cos(q2))^2 + 2 * J13 * cos(q2) * sin(q2+q3);
h22 = J1 + J12 + 2 * J13 * sin(q3);
h23 = J1 + J13 * sin(q3);
h32 = h23;
h33 = J1;

H = [h11, 0 ,0 ;
    0 , h22, h23;
    0 , h32, h33];

%% Coriolis Matrix Parameters

c12_1 = J1 * sin(2 * (q1 + q2)) - J12 * sin(2 * q2) + 2 * J13 * cos(2 * q2 +q3);
c13_1 = J1 * sin(2 * (q2 + q3)) + 2 * J13 * cos(q2) * cos(q2 + q3);
c11_2 = (1/2) * (-J1 * sin(2 * (q2 + q3)) + J12 * sin(2 * q2) - 2 * J13 * cos(2 * q2 + q3));
c22_2 = 2 * J13 * cos(q3);
c23_2 = J13 * cos(q3);
c22_3 = -J13 * cos(q3) * dq2;
c11_3 = (-1/2) * (J1 * sin(2 * (q2 + q3)) + J13 * cos(q2) * cos(q2 + q3));

C = [0, c12_1 * dq1, c13_1 * dq3;
    c11_2 * dq1, 0 , c22_2 * dq2 + c23_2 * dq3;
    c11_3 * dq1, c22_3 * dq2, 0];

%% Vector of Potential Forces Parameters

g = 9.81;

g21 = -g * (lc3 * m3 * sin(q2 + q3) + lc2 * m2 * cos(q2) + l2 * m3 * cos(q2));
g31 = -g * (lc3 * m3 * sin(q2 + q3));

G = [0;
    g21;
    g31];

%% Function output

ddq = inv(H)*(tau + tau_e - C * dq - G);

== matlab function best_project_for_IG/FWDKinematics3/MATLAB Function ==
  data: q input; X output
function X = FWDKinematics(q)
%%% Forward Kinematic Function


%% Joint Space variables
% q is 3*1 vector of joint variables (radian), q = [q1;q2;q3]
q1 = q(1);
q2 = q(2);
q3 = q(3);

%% general physical parameters
l1 = 0.6731;
l2 = 0.432;
l3 = 0.434;
lc2 = 0.216;
lc3 = 0.164;

%% Forward Kinematic
% X is 3*1 vecto of end-effector position in task space, X = [x;y;z]

x = cos(q1) * (l2 * cos(q2) + l3 * sin(q2 + q3));
y = sin(q1) * (l2 * cos(q2) + l3 * sin(q2 + q3));
z = l1 - l2 * sin(q2) + l3 * cos(q2 + q3);

X = [x;y;z];

== matlab function best_project_for_IG/Robot 1: Manipulator Dynamic/MATLAB Function ==
  data: tau input; tau_e input; q input; ddq output; dq input
function ddq = DynamicModel( tau, tau_e, q, dq)
%%%%%
% 3-DOF Puma-560 Dynamic Model Function
% H(q)* ddq + C(q) * dq + G = tau + tau_e
% q is 3*1 vector of joint variables (radian)
% H(q) is the inertia matrix
% C(q) is the matrix of Coriolis and centrifugal forces
% G(q) is  the vector of potential forces Parameters
% tau is control torque 
% tau_e is the external torque due to the interaction with the environment
%%%%%

%% Joint Space variables

q1 = q(1);
q2 = q(2);
q3 = q(3);

dq1 = dq(1);
dq2 = dq(2);
dq3 = dq(3);

%% general physical parameters

l1 = 0.6731;
l2 = 0.432;
l3 = 0.434;
lc2 = 0.216;
lc3 = 0.164;
m2 = 15.46;
m3 = 9.55;
J = 0.302;

%% Inertia Matrix Parameters

J1 = m3 * lc3^2;
J12 = (m2 * lc2^2) + (m3 * l2^2);
J13 = l2 * lc3 * m3;


h11 = J + J1 * (sin(q2 + q3))^2 + J12 * (cos(q2))^2 + 2 * J13 * cos(q2) * sin(q2+q3);
h22 = J1 + J12 + 2 * J13 * sin(q3);
h23 = J1 + J13 * sin(q3);
h32 = h23;
h33 = J1;

H = [h11, 0 ,0 ;
    0 , h22, h23;
    0 , h32, h33];

%% Coriolis Matrix Parameters

c12_1 = J1 * sin(2 * (q1 + q2)) - J12 * sin(2 * q2) + 2 * J13 * cos(2 * q2 +q3);
c13_1 = J1 * sin(2 * (q2 + q3)) + 2 * J13 * cos(q2) * cos(q2 + q3);
c11_2 = (1/2) * (-J1 * sin(2 * (q2 + q3)) + J12 * sin(2 * q2) - 2 * J13 * cos(2 * q2 + q3));
c22_2 = 2 * J13 * cos(q3);
c23_2 = J13 * cos(q3);
c22_3 = -J13 * cos(q3) * dq2;
c11_3 = (-1/2) * (J1 * sin(2 * (q2 + q3)) + J13 * cos(q2) * cos(q2 + q3));

C = [0, c12_1 * dq1, c13_1 * dq3;
    c11_2 * dq1, 0 , c22_2 * dq2 + c23_2 * dq3;
    c11_3 * dq1, c22_3 * dq2, 0];

%% Vector of Potential Forces Parameters

g = 9.81;

g21 = -g * (lc3 * m3 * sin(q2 + q3) + lc2 * m2 * cos(q2) + l2 * m3 * cos(q2));
g31 = -g * (lc3 * m3 * sin(q2 + q3));

G = [0;
    g21;
    g31];

%% Function output

ddq = inv(H)*(tau + tau_e - C * dq - G);

== matlab function best_project_for_IG/FWDKinematics2/MATLAB Function ==
  data: q input; X output
function X = FWDKinematics(q)
%%% Forward Kinematic Function


%% Joint Space variables
% q is 3*1 vector of joint variables (radian), q = [q1;q2;q3]
q1 = q(1);
q2 = q(2);
q3 = q(3);

%% general physical parameters
l1 = 0.6731;
l2 = 0.432;
l3 = 0.434;
lc2 = 0.216;
lc3 = 0.164;

%% Forward Kinematic
% X is 3*1 vecto of end-effector position in task space, X = [x;y;z]

x = cos(q1) * (l2 * cos(q2) + l3 * sin(q2 + q3));
y = sin(q1) * (l2 * cos(q2) + l3 * sin(q2 + q3));
z = l1 - l2 * sin(q2) + l3 * cos(q2 + q3);

X = [x;y;z];

== matlab function best_project_for_IG/R2 Impedence Controller/MATLAB Function ==
  data: q input; dq input; ddq input; tau_control output; qd input; qd_dot input; qd_ddot input; force input; time input; Hm_const input; Dm_const input; Km_const input
function tau_control = fcn(q, dq, ddq, qd, qd_dot, qd_ddot,force,...
                           time, Hm_const, Dm_const, Km_const)
% reset first qd_ddot
if (time < 0.003)
    qd_ddot = [0;0;0];
    qd_dot = [0;0;0];
    ddq = [0;0;0];
end


%% Joint Space variables

q1 = q(1);
q2 = q(2);
q3 = q(3);

dq1 = dq(1);
dq2 = dq(2);
dq3 = dq(3);

%% general physical parameters

l1 = 0.6731;
l2 = 0.432;
l3 = 0.434;
lc2 = 0.216;
lc3 = 0.164;
m2 = 15.46;
m3 = 9.55;
J = 0.302;

%% Inertia Matrix Parameters

J1 = m3 * lc3^2;
J12 = (m2 * lc2^2) + (m3 * l2^2);
J13 = l2 * lc3 * m3;


h11 = J + J1 * (sin(q2 + q3))^2 + J12 * (cos(q2))^2 + 2 * J13 * cos(q2) * sin(q2+q3);
h22 = J1 + J12 + 2 * J13 * sin(q3);
h23 = J1 + J13 * sin(q3);
h32 = h23;
h33 = J1;

H = [h11, 0 ,0 ;
    0 , h22, h23;
    0 , h32, h33];

%% Coriolis Matrix Parameters

c12_1 = J1 * sin(2 * (q1 + q2)) - J12 * sin(2 * q2) + 2 * J13 * cos(2 * q2 +q3);
c13_1 = J1 * sin(2 * (q2 + q3)) + 2 * J13 * cos(q2) * cos(q2 + q3);
c11_2 = (1/2) * (-J1 * sin(2 * (q2 + q3)) + J12 * sin(2 * q2) - 2 * J13 * cos(2 * q2 + q3));
c22_2 = 2 * J13 * cos(q3);
c23_2 = J13 * cos(q3);
c22_3 = -J13 * cos(q3) * dq2;
c11_3 = (-1/2) * (J1 * sin(2 * (q2 + q3)) + J13 * cos(q2) * cos(q2 + q3));

C = [0, c12_1 * dq1, c13_1 * dq3;
    c11_2 * dq1, 0 , c22_2 * dq2 + c23_2 * dq3;
    c11_3 * dq1, c22_3 * dq2, 0];

%% Vector of Potential Forces Parameters

g = 9.81;

g21 = -g * (lc3 * m3 * sin(q2 + q3) + lc2 * m2 * cos(q2) + l2 * m3 * cos(q2));
g31 = -g * (lc3 * m3 * sin(q2 + q3));

G = [0;
    g21;
    g31];


%% get Jacobians
J = jacobian(q);
dJ = dJacobian(q,dq);

%% convert to task space
Hp = inv(J') * H * inv(J);
Cp = inv(J') * C * inv(J) - Hp * dJ * inv(J);
Gp = inv(J') * G;

%% desired behaviour
Hm = Hm_const*eye(3,3);
Dm = Dm_const*eye(3,3);
Km = Km_const*eye(3,3);

%% get postion and its derivs
p = fwdKin(q);
dp = J * dq;
ddp = dJ * dq + J * ddq;

%% get desired postion and its derivs
pd = fwdKin(qd);
pd_dot = jacobian(qd) * qd_dot;
pd_ddot = dJacobian(qd,qd_dot) * qd_dot + jacobian(qd) * qd_ddot;

%% define u note

u_note = pd_ddot + inv(Hm) * (Dm * (pd_dot-dp) + Km*(pd - p) + force);
inv_hm = inv(Hm);
%% define tau_control

tau_control = J' * (Hp * u_note + Cp * dp + Gp - force);


function [X] = fwdKin(Q)
    s1 = sin(Q(1, :));
    c1 = cos(Q(1, :));
    s2 = sin(Q(2, :));
    c2 = cos(Q(2, :));
    s23 = sin(Q(2, :) + Q(3, :));
    c23 = cos(Q(2, :) + Q(3, :));
    l = [0.6731; 0.432; 0.434];
    
    X = zeros(3,1);
    X(1, :) = c1.*(l(2)*c2 + l(3)*s23);
    X(2, :) = s1.*(l(2)*c2 + l(3)*s23);
    X(3, :) = l(1) - l(2)*s2 + l(3)*c23;

function dJ = dJacobian(Q, dQ)
    l = [0.6731; 0.432; 0.434];
    s1 = sin(Q(1));
    c1 = cos(Q(1));
    s2 = sin(Q(2));
    c2 = cos(Q(2));
    s23 = sin(Q(2) + Q(3));
    c23 = cos(Q(2) + Q(3));

    % dJi derivative of each element of Jacobian wrt i-th variable            
    %--- 1 ---
    dJ1 = [-c1*(l(2)*c2 + l(3)*s23), -s1*(-l(2)*s2 + l(3)*c23), -l(3)*s1*c23;...
           -s1*(l(2)*c2 + l(3)*s23),  c1*(-l(2)*s2 + l(3)*c23),  l(3)*c1*c23;...
           0, 0, 0];
    %--- 2 ---   
    dJ2 = [-s1*(-l(2)*s2 + l(3)*c23), -c1*(l(2)*c2 + l(3)*s23), -l(3)*c1*s23;...
            c1*(-l(2)*s2 + l(3)*c23), -s1*(l(2)*c2 + l(3)*s23), -l(3)*s1*s23;...
            0, l(2)*s2 - l(3)*c23, -l(3)*c23];

    %--- 3 ---
    dJ3 = -l(3)*[ s1*c23, c1*s23, c1*s23;...
                 -c1*c23, s1*s23, s1*s23;...
                 0, c23, c23];
    %--- dJ ---
    dJ = dJ1*dQ(1) + dJ2*dQ(2) + dJ3*dQ(3);

function [J] = jacobian(q)

l = [0.6731; 0.432; 0.434];
s1 = sin(q(1));
c1 = cos(q(1));
s2 = sin(q(2));
c2 = cos(q(2));
s23 = sin(q(2) + q(3));
c23 = cos(q(2) + q(3));

J = zeros(3,3);

J(1, 1) = -s1*( l(2)*c2 + l(3)*s23);
J(1, 2) =  c1*(-l(2)*s2 + l(3)*c23);
J(1, 3) = l(3)*c1*c23;

J(2, 1) = c1*( l(2)*c2 + l(3)*s23);
J(2, 2) = s1*(-l(2)*s2 + l(3)*c23);
J(2, 3) = l(3)*s1*c23;

J(3, 2) = -l(2)*c2 - l(3)*s23;
J(3, 3) = -l(3)*s23;

== matlab function best_project_for_IG/MATLAB Function ==
  data: time input; R1_des_pose input; R1_pose input; R1_velocity input; time_offset input; time_offset output; is_triggered input; is_triggered output
function [time_offset, is_triggered] = fcn(time, R1_des_pose, R1_pose, R1_velocity, time_offset, is_triggered)

if ((time > 6 && ...
        norm(R1_des_pose - R1_pose) <= 0.1 && ...
        norm(R1_velocity) <= 0.002) && (is_triggered==0))
    time_offset = time;
    is_triggered = 1;
end
